simulink model "Plant_sim"  (R2023a)
settings: Solver=FixedStepAuto  StartTime=0.0  StopTime=10  FixedStep=0.001  RelTol=1e-3
values from neighbouring files (symbols this model uses):
  A = d_sys.A    [DiscreteKalmanFilter.m]
  b = 4.37E-4    (= 0.000437)    [DiscreteKalmanFilter.m]
  B = d_sys.B    [DiscreteKalmanFilter.m]
  C = d_sys.C    [DiscreteKalmanFilter.m]
  D = d_sys.D    [DiscreteKalmanFilter.m]
  G = Gc    [DiscreteKalmanFilter.m]
  J = 1.7E-6    (= 1.7e-06)    [DiscreteKalmanFilter.m]
  ke = (3.65e-3)/60    (= 6.08333333333e-05)    [DiscreteKalmanFilter.m]
  kt = 34.8E-3    (= 0.0348)    [DiscreteKalmanFilter.m]
  L = 380E-6    (= 0.00038)    [DiscreteKalmanFilter.m]
  R = 1    [DiscreteKalmanFilter.m]
undefined symbols (not defined in the file or in its folder): DiscIntNeverNeededParam, Discrete, Time
libraries: simulink x2, ctrlSharedLib x1, robotcorelib x1
settings Model: Creator=pawee  LastModifiedBy=User
settings DebuggingCC: UnderSpecifiedDimensionMsg=warning
settings ModelReferenceCC: EnableRefExpFcnMdlSchedulingChecks=on

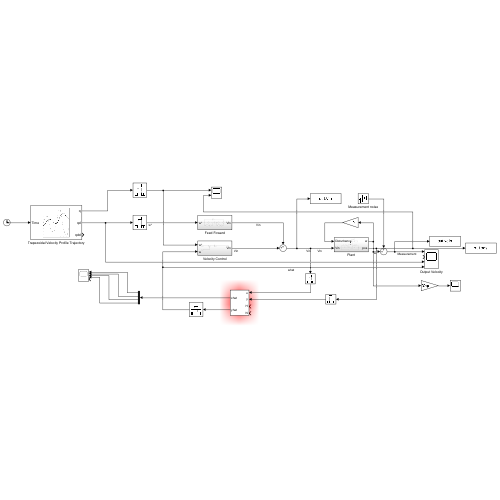
[thumbnail: Simulink's stored preview of the top-level diagram]
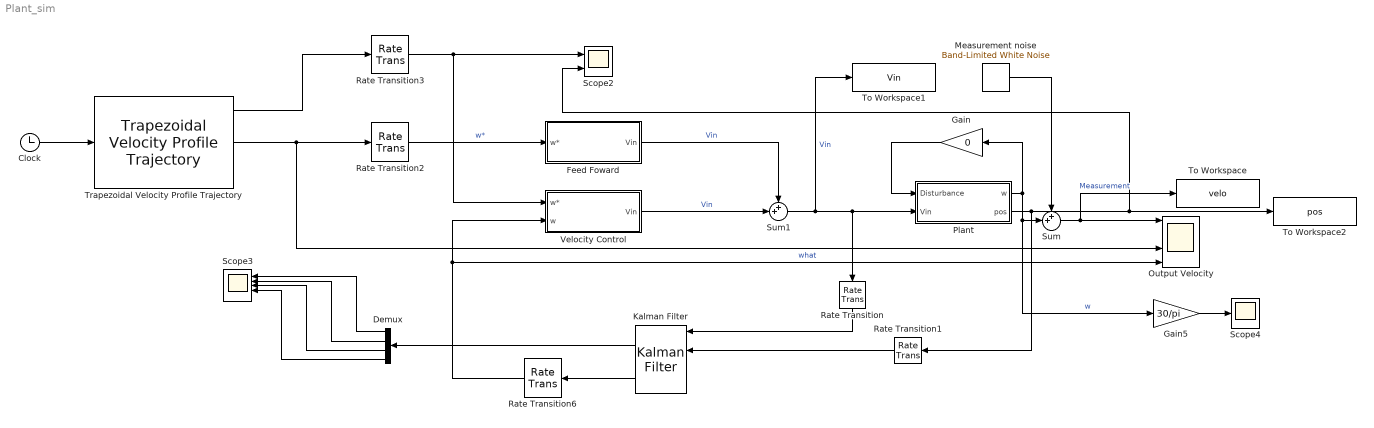
== system Plant_sim ==
  Clock : Clock
  Demux : Demux
  Feed Foward : Subsystem
  Gain : Gain  Gain=0
  Gain5 : Gain  Gain=30/pi
  Kalman Filter : ctrlSharedLib/Kalman Filter  TimeDomain=Discrete-Time  UseCurrentEstimator=on  ModelSource=Individual A, B, C, D matrices  ModelSourceVariable=ss(0.95,1,1,0,1)  A=A  B=B  C=C  D=D  NumberOfStates=1  NumberOfInputs=1  NumberOfOutputs=1  InitialEstimateSource=Dialog  X0=0  P0=1  UseK=off  UseGH=on  NumberOfProcessNoiseInputs=1  G=G  TimeInvariantG=on  H=0  TimeInvariantH=off  Q=1  TimeInvariantQ=on  R=99999  TimeInvariantR=on  N=G  TimeInvariantN=off  AddInputPort=on  AddEnablePort=off  OutputEstimatedY=on  OutputP=off  Ts=-1
  Measurement noise : simulink/Sources/Band-Limited White Noise  Cov=[0.1]  Ts=0.01  seed=[23341]
  Output Velocity : Scope  NumInputPorts=4
  Plant : Subsystem
  Rate Transition : RateTransition  OutPortSampleTimeOpt=Inherit  OutPortSampleTimeMultiple=0
  Rate Transition1 : RateTransition  OutPortSampleTimeOpt=Inherit  OutPortSampleTimeMultiple=0
  Rate Transition2 : RateTransition  OutPortSampleTimeOpt=Inherit
  Rate Transition3 : RateTransition  OutPortSampleTimeOpt=Inherit
  Rate Transition6 : RateTransition  OutPortSampleTimeOpt=Inherit
  Scope2 : Scope  NumInputPorts=2
  Scope3 : Scope  NumInputPorts=5
  Scope4 : Scope
  Sum : Sum  Inputs=++|
  Sum1 : Sum  Inputs=++|
  To Workspace : ToWorkspace  VariableName=velo  SaveFormat=Timeseries  SampleTime=-1
  To Workspace1 : ToWorkspace  VariableName=Vin  SaveFormat=Timeseries  SampleTime=-1
  To Workspace2 : ToWorkspace  VariableName=pos  SaveFormat=Timeseries  SampleTime=-1
  Trapezoidal Velocity Profile Trajectory : robotcorelib/Trapezoidal Velocity Profile Trajectory  WaypointSource=Internal  Waypoints=[ 0, 70, 300]  NumParams=2  Parameter1=Peak Velocity  Parameter2=Acceleration  ParameterSource=Internal  PeakVelocity=[50]  Acceleration=[60]  EndTime=[ 1; 1 ]  AccelTime=[ 1; 2 ]  SimulateUsing=Interpreted execution
  Velocity Control : Subsystem
  wires:
  Clock/1 -> Trapezoidal Velocity Profile Trajectory/1
  Sum/1 -> To Workspace/1, Output Velocity/1  "Measurement"
  Measurement noise/1 -> Sum/1
  Feed Foward/1(Vin) -> Sum1/1  "Vin"
  Gain/1 -> Plant/1(Disturbance)
  Plant/1(w) -> Gain5/1, Sum/2, Gain/1  "w"
  Rate Transition/1 -> Kalman Filter/1
  Rate Transition2/1 -> Feed Foward/1(w*)  "w*"
  Trapezoidal Velocity Profile Trajectory/1 -> Rate Transition3/1
  Kalman Filter/2 -> Rate Transition6/1
  Velocity Control/1(Vin) -> Sum1/2  "Vin"
  Rate Transition6/1 -> Velocity Control/2(w), Output Velocity/4  "what"
  Rate Transition3/1 -> Scope2/1, Velocity Control/1(w*)
  Trapezoidal Velocity Profile Trajectory/2 -> Output Velocity/3, Rate Transition2/1
  Rate Transition1/1 -> Kalman Filter/2
  Sum1/1 -> To Workspace1/1, Plant/2(Vin), Rate Transition/1  "Vin"
  Plant/2(pos) -> Rate Transition1/1, To Workspace2/1, Scope2/2
  Kalman Filter/1 -> Demux/1
  Demux/2 -> Scope3/2
  Demux/1 -> Scope3/1
  Demux/3 -> Scope3/3
  Demux/4 -> Scope3/4
  Gain5/1 -> Scope4/1

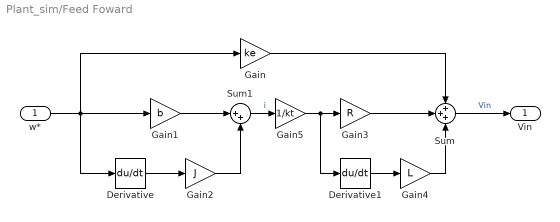
== system Plant_sim/Feed Foward ==
  w* : Inport
  Derivative : Derivative
  Derivative1 : Derivative
  Gain : Gain  Gain=ke
  Gain1 : Gain  Gain=b
  Gain2 : Gain  Gain=J
  Gain3 : Gain  Gain=R
  Gain4 : Gain  Gain=L
  Gain5 : Gain  Gain=1/kt
  Sum : Sum  Inputs=+++
  Sum1 : Sum  Inputs=|++
  Vin : Outport
  wires:
  w*/1 -> Gain/1, Derivative/1, Gain1/1
  Gain3/1 -> Sum/2
  Gain/1 -> Sum/1
  Sum/1 -> Vin/1  "Vin"
  Gain1/1 -> Sum1/1
  Derivative/1 -> Gain2/1
  Gain2/1 -> Sum1/2
  Derivative1/1 -> Gain4/1
  Gain4/1 -> Sum/3
  Sum1/1 -> Gain5/1  "i"
  Gain5/1 -> Derivative1/1, Gain3/1

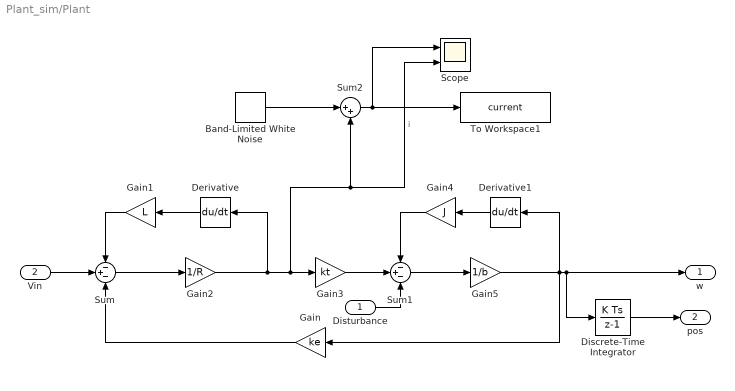
== system Plant_sim/Plant ==
  Disturbance : Inport
  Vin : Inport  Port=2
  Band-Limited White Noise : simulink/Sources/Band-Limited White Noise  Cov=[0.001]  Ts=0.01  seed=[23341]
  Derivative : Derivative
  Derivative1 : Derivative
  Discrete-Time Integrator : DiscreteIntegrator  SampleTime=-1  ICPrevOutput=DiscIntNeverNeededParam  ICPrevScaledInput=DiscIntNeverNeededParam
  Gain : Gain  Gain=ke
  Gain1 : Gain  Gain=L
  Gain2 : Gain  Gain=1/R
  Gain3 : Gain  Gain=kt
  Gain4 : Gain  Gain=J
  Gain5 : Gain  Gain=1/b
  Scope : Scope  NumInputPorts=2
  Sum : Sum  Inputs=-+-
  Sum1 : Sum  Inputs=-+-
  Sum2 : Sum  Inputs=|++
  To Workspace1 : ToWorkspace  VariableName=current  SaveFormat=Timeseries  SampleTime=-1
  w : Outport
  pos : Outport  Port=2
  wires:
  Sum/1 -> Gain2/1
  Gain/1 -> Sum/3
  Vin/1 -> Sum/2
  Gain1/1 -> Sum/1
  Derivative/1 -> Gain1/1
  Gain2/1 -> Derivative/1, Sum2/2, Scope/2, Gain3/1  "i"
  Derivative1/1 -> Gain4/1
  Gain4/1 -> Sum1/1
  Gain5/1 -> Discrete-Time Integrator/1, w/1, Gain/1, Derivative1/1
  Disturbance/1 -> Sum1/3
  Gain3/1 -> Sum1/2
  Discrete-Time Integrator/1 -> pos/1
  Band-Limited White Noise/1 -> Sum2/1
  Sum2/1 -> Scope/1, To Workspace1/1
  Sum1/1 -> Gain5/1

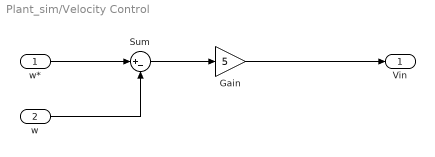
== system Plant_sim/Velocity Control ==
  w* : Inport
  w : Inport  Port=2
  Gain : Gain  Gain=5
  Sum : Sum  Inputs=|+-
  Vin : Outport
  wires:
  w*/1 -> Sum/1
  w/1 -> Sum/2
  Sum/1 -> Gain/1
  Gain/1 -> Vin/1
